simulink model "test"  (R2016b)
settings: Solver=VariableStepAuto  StartTime=0.0  StopTime=10  RelTol=1e-3
settings Model: Creator=96919  LastModifiedBy=96919

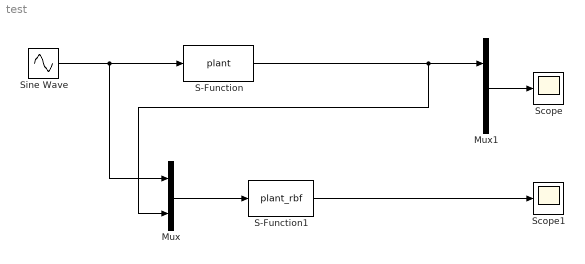
== system test ==
  Mux : Mux  Inputs=2
  Mux1 : Mux  Inputs=2
  S-Function : S-Function  FunctionName=plant  SFunctionDeploymentMode=off  EnableBusSupport=off
  S-Function1 : S-Function  FunctionName=plant_rbf  SFunctionDeploymentMode=off  EnableBusSupport=off
  Scope : Scope
  Scope1 : Scope
  Sine Wave : Sin  SampleTime=0
  wires:
  Sine Wave/1 -> Mux/1, S-Function/1
  S-Function/1 -> Mux1/1, Mux/2
  Mux/1 -> S-Function1/1
  Mux1/1 -> Scope/1
  S-Function1/1 -> Scope1/1
